simulink model "ventilation"  (R2020a)
settings: Solver=FixedStepAuto  StartTime=0.0  StopTime=25  RelTol=1e-3
undefined symbols (not defined in the file): Ci, Pex, Pset, Ri, T, ti, Ve0, Vt
libraries: dspswit3 x1
settings Model: Creator=sebastian  LastModifiedBy=luisi
settings OptimizationCC: EnhancedBackFolding=on  PassReuseOutputArgsAs=Individual arguments  ZeroExternalMemoryAtStartup=off  ZeroInternalMemoryAtStartup=off  MaxStackSize=64  OptimizeBlockOrder=speed  DifferentSizesBufferReuse=on  OptimizationCustomize=off  EfficientTunableParamExpr=on
settings DebuggingCC: ParameterTunabilityLossMsg=error
settings HardwareCC: ProdBitPerPointer=32  ProdBitPerSizeT=32  ProdBitPerPtrDiffT=32  ProdLargestAtomicInteger=Long  ProdLargestAtomicFloat=Double  ProdWordSize=32  ProdHWDeviceType=ARM Compatible->ARM Cortex
settings SFSimCC: MATLABDynamicMemAlloc=off
settings RTWCC: SystemTargetFile=ert.tlc  HardwareBoard=Android Device  TemplateMakefile=ert_default_tmf  RTWVerbose=off  Toolchain=Android SDK/NDK Tools
settings CodeAppCC: ForceParamTrailComments=on  IgnoreCustomStorageClasses=off  OperatorAnnotations=on  SimulinkDataObjDesc=on  SFDataObjDesc=on  InsertBlockDesc=on
settings ERTTargetCC: SupportContinuousTime=on

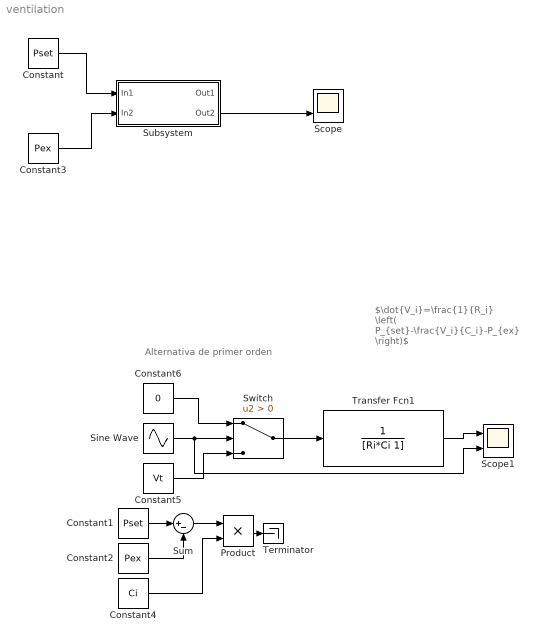
== system ventilation ==
  note: Alternativa de primer orden
  note: $\dot{V_i}=\frac{1}{R_i} \left( P_{set}-\frac{V_i}{C_i}-P_{ex} \right)$
  Constant : Constant  Value=Pset
  Constant1 : Constant  Value=Pset
  Constant2 : Constant  Value=Pex
  Constant3 : Constant  Value=Pex
  Constant4 : Constant  Value=Ci
  Constant5 : Constant  Value=Vt
  Constant6 : Constant  Value=0
  Product : Product
  Scope : Scope  NumInputPorts=2
  Scope1 : Scope  NumInputPorts=2
  Sine Wave : Sin  Frequency=0.5*pi  SampleTime=0
  Subsystem : Subsystem
  Sum : Sum  Inputs=|+-
  Switch : Switch  Criteria=u2 > Threshold
  Terminator : Terminator
  Transfer Fcn1 : TransferFcn  Denominator=[Ri*Ci 1]
  wires:
  Constant/1 -> Subsystem/1(In1)
  Constant3/1 -> Subsystem/2(In2)
  Subsystem/2(Out2) -> Scope/2
  Constant1/1 -> Sum/1
  Constant2/1 -> Sum/2
  Sum/1 -> Product/1
  Constant4/1 -> Product/2
  Constant6/1 -> Switch/1
  Switch/1 -> Transfer Fcn1/1
  Transfer Fcn1/1 -> Scope1/1
  Sine Wave/1 -> Scope1/2, Switch/2
  Constant5/1 -> Switch/3
  Product/1 -> Terminator/1

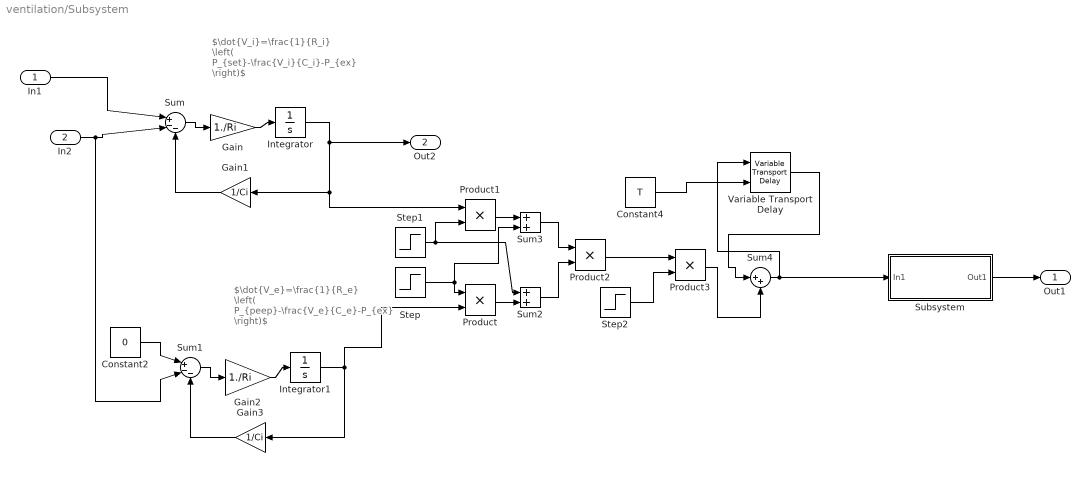
== system ventilation/Subsystem ==
  note: $\dot{V_i}=\frac{1}{R_i} \left( P_{set}-\frac{V_i}{C_i}-P_{ex} \right)$
  note: $\dot{V_e}=\frac{1}{R_e} \left( P_{peep}-\frac{V_e}{C_e}-P_{ex} \right)$
  In1 : Inport
  In2 : Inport  Port=2
  Constant2 : Constant  Value=0
  Constant4 : Constant  Value=T
  Gain : Gain  Gain=1./Ri
  Gain1 : Gain  Gain=1/Ci
  Gain2 : Gain  Gain=1./Ri
  Gain3 : Gain  Gain=1/Ci
  Integrator : Integrator
  Integrator1 : Integrator  InitialCondition=Ve0
  Product{,1..3} (4 alike) : Product
  Step : Step  Time=ti  SampleTime=0
  Step1 : Step  Time=ti  Before=1  After=0  SampleTime=0
  Step2 : Step  Time=T  Before=1  After=0  SampleTime=0
  Subsystem : Subsystem
  Sum : Sum  Inputs=|+--
  Sum1 : Sum  Inputs=|+--
  Sum2 : Sum
  Sum3 : Sum
  Sum4 : Sum  Inputs=|++
  Variable Transport Delay : VariableTransportDelay  VariableDelayType=Variable transport delay  MaximumDelay=10
  Out1 : Outport
  Out2 : Outport  Port=2
  wires:
  Sum3/1 -> Product2/1
  Constant4/1 -> Variable Transport Delay/2
  Sum2/1 -> Product2/2
  Gain3/1 -> Sum1/3
  Integrator1/1 -> Product/2, Gain3/1
  Product2/1 -> Product3/1
  Product1/1 -> Sum3/1
  Step2/1 -> Product3/2
  Product3/1 -> Sum4/2
  Integrator/1 -> Product1/1, Gain1/1, Out2/1
  Step/1 -> Product/1, Sum3/2
  Product/1 -> Sum2/2
  Sum4/1 -> Variable Transport Delay/1, Subsystem/1(In1)
  Gain2/1 -> Integrator1/1
  Variable Transport Delay/1 -> Sum4/1
  Gain1/1 -> Sum/3
  Subsystem/1(Out1) -> Out1/1
  Sum1/1 -> Gain2/1
  Step1/1 -> Sum2/1, Product1/2
  In2/1 -> Sum1/2, Sum/2
  Constant2/1 -> Sum1/1
  Gain/1 -> Integrator/1
  Sum/1 -> Gain/1
  In1/1 -> Sum/1

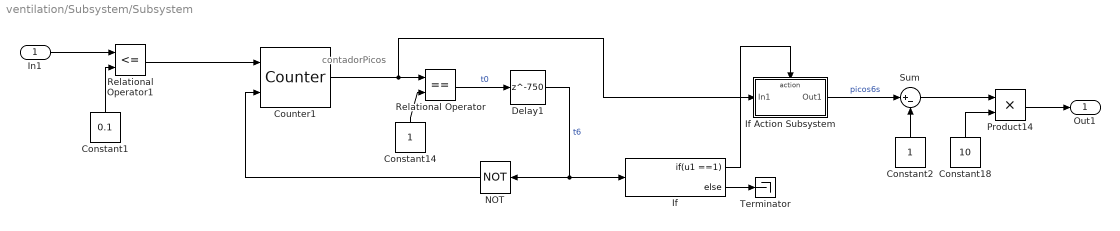
== system ventilation/Subsystem/Subsystem ==
  note: contadorPicos
  In1 : Inport
  Constant1 : Constant  Value=0.1
  Constant14 : Constant
  Constant18 : Constant  Value=10
  Constant2 : Constant
  Counter1 : dspswit3/Counter  Direction=Up  CountEvent=Rising edge  CounterSize=User defined  MaxCount=100  InitialCount=0  Output=Count  HitValue=32  ResetInput=on  SamplesPerFrame=1  Ts=1  CntDtype=double  HitDtype=Logical
  Delay1 : Delay  DelayLength=750  SampleTime=0.008
  If : If  IfExpression=u1 ==1
  If Action Subsystem : Subsystem  TreatAsAtomicUnit=on
  NOT : Logic  Operator=NOT  IconShape=distinctive  AllPortsSameDT=off  OutDataTypeStr=boolean
  Product14 : Product
  Relational Operator : RelationalOperator  Operator===  OutDataTypeStr=boolean  RndMeth=Simplest
  Relational Operator1 : RelationalOperator  Operator=<=  OutDataTypeStr=boolean  RndMeth=Simplest
  Sum : Sum  Inputs=|+-
  Terminator : Terminator
  Out1 : Outport
  wires:
  Relational Operator1/1 -> Counter1/1
  Relational Operator/1 -> Delay1/1  "t0"
  Product14/1 -> Out1/1
  If/2 -> Terminator/1
  Constant18/1 -> Product14/2
  Delay1/1 -> NOT/1, If/1  "t6"
  NOT/1 -> Counter1/2
  In1/1 -> Relational Operator1/1
  Counter1/1 -> If Action Subsystem/1(In1), Relational Operator/1
  If/1 -> If Action Subsystem/Action
  Constant14/1 -> Relational Operator/2
  Constant1/1 -> Relational Operator1/2
  If Action Subsystem/1(Out1) -> Sum/1  "picos6s"
  Sum/1 -> Product14/1
  Constant2/1 -> Sum/2

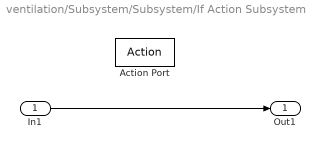
== system ventilation/Subsystem/Subsystem/If Action Subsystem ==
  In1 : Inport
  Action Port : ActionPort  ActionPortLabel=if(u1 ==1)
  Out1 : Outport
  wires:
  In1/1 -> Out1/1
